simulink model "sim_3_twolink_task_control"  (R2021a)
settings: Solver=VariableStepAuto  StartTime=0.0  StopTime=10.0  RelTol=1e-3
values from neighbouring files (symbols this model uses):
  b1 = 0.01    [sim_params.m]    (also in sim_params_force.m)
  b2 = 0.01    [sim_params.m]    (also in sim_params_force.m)
  D = [zeros(n); eye(n)]    [control_comparison_script.m]    (also in gen_twolink_ss.m = reshape([0.0,0.0,0.0,0.0,0.0,0.0,0.0,0.0],[4,2]))
  g = 9.80665    [sim_params.m]    (also in sim_params_force.m)
  Klqr = lqr(A,B,Q,R)    [control_comparison_script.m]
  Kpp = place(A,B,p)    [control_comparison_script.m]
  L1x = 0.3    [sim_params.m]    (also in sim_params_force.m)
  L1y = 0.050    (= 0.05)    [sim_params.m]    (also in sim_params_force.m)
  L1z = 0.05    [sim_params.m]    (also in sim_params_force.m)
  L2x = 0.15    [sim_params.m]    (also in sim_params_force.m = 0.3)
  L2y = 0.05    [sim_params.m]    (also in sim_params_force.m)
  L2z = 0.05    [sim_params.m]    (also in sim_params_force.m)
  m1 = m1*1.25    [control_comparison_script.m]    (also in sim_params.m = 2.775; sim_params_force.m = 2.775)
  m2 = m2*1.25    [control_comparison_script.m]    (also in sim_params.m = 1.3875; sim_params_force.m = 2.775)
  max_joint_torque1 = 20    [sim_params.m]    (also in sim_params_force.m)
  max_joint_torque2 = 10    [sim_params.m]    (also in sim_params_force.m = 20)
  theta1_0 = 0    [sim_params.m]    (also in sim_params_force.m = 1.57079632679)
  theta1_dot_0 = 0    [sim_params.m]    (also in sim_params_force.m)
  theta2_0 = 0    [sim_params.m]    (also in sim_params_force.m = -1.57079632679)
  theta2_dot_0 = 0    [sim_params.m]    (also in sim_params_force.m)
undefined symbols (not defined in the file or in its folder): Kslide, lambda, Levenberg, Marquardt, phi, sigbuilder_block, X, Y, Z
libraries: sm_lib x11, nesl_utility x10, simulink x8, pid_lib x6, robotmaniplib x3, robotcorelib x1
(part 2 of 2)

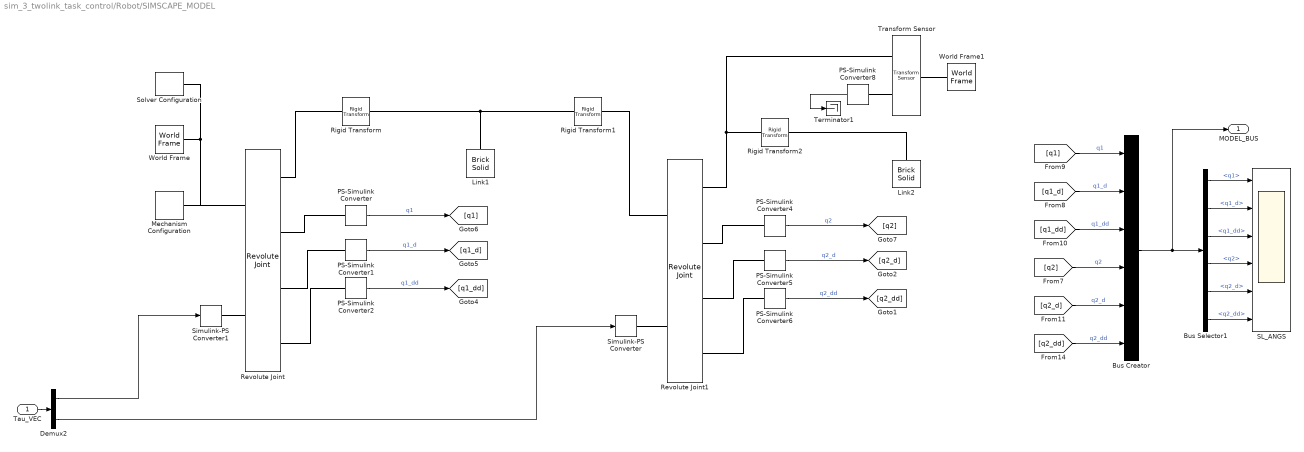
== system sim_3_twolink_task_control/Robot/SIMSCAPE_MODEL ==
  Tau_VEC : Inport
  Bus Creator : BusCreator  Inputs=6
  Bus Selector1 : BusSelector  OutputSignals=q1,q1_d,q1_dd,q2,q2_d,q2_dd
  Demux2 : Demux  Outputs=2
  Link1 : sm_lib/Body Elements/Brick Solid  GraphicAmbientColor=[0.15 0.15 0.15 1.0]  BasedOnType=Density  BrickDimensions=[L1x L1y L1z]  BrickDimensionUnits=m  CenterOfMass=[0 0 0]  CenterOfMassUnits=m  GraphicDiffuseColor=[0.8 0.8 1.0]  Density=density  DensityUnits=kg/m^3  DoExposeReferenceFrame=on  GraphicEmissiveColor=[0.0 0.0 0.0 1.0]  ExportEntireGeometry=off  SerializedFrames=<Frames/>  MarkerShape=Sphere  MarkerSize=10  GraphicType=FromGeometry  InertiaType=CalculateFromGeometry  Mass=1  MassUnits=kg  MomentsOfInertia=[1 1 1]  MomentsOfInertiaUnits=kg*m^2  GraphicOpacity=1.0  ProductsOfInertia=[0 0 0]  ProductsOfInertiaUnits=kg*m^2  GraphicShininess=75  GraphicSpecularColor=[0.5 0.5 0.5 1.0]  GraphicVisPropType=SimpleVisualProperties
  Link2 : sm_lib/Body Elements/Brick Solid  GraphicAmbientColor=[0.15 0.15 0.15 1.0]  BasedOnType=Density  BrickDimensions=[L2x L2y L2z]  BrickDimensionUnits=m  CenterOfMass=[0 0 0]  CenterOfMassUnits=m  GraphicDiffuseColor=[1.0 0.6 1.0]  Density=density  DensityUnits=kg/m^3  DoExposeReferenceFrame=on  GraphicEmissiveColor=[0.0 0.0 0.0 1.0]  ExportEntireGeometry=off  SerializedFrames=<Frames/>  MarkerShape=Sphere  MarkerSize=10  GraphicType=FromGeometry  InertiaType=CalculateFromGeometry  Mass=1  MassUnits=kg  MomentsOfInertia=[1 1 1]  MomentsOfInertiaUnits=kg*m^2  GraphicOpacity=1.0  ProductsOfInertia=[0 0 0]  ProductsOfInertiaUnits=kg*m^2  GraphicShininess=75  GraphicSpecularColor=[0.5 0.5 0.5 1.0]  GraphicVisPropType=SimpleVisualProperties
  Mechanism Configuration : sm_lib/Utilities/Mechanism Configuration  UniformGravity=Constant  GravityVector=[0 -g 0 ]  GravityVectorUnits=m/s^2  GravityUnits=m/s^2  LinearizationDelta=1e-4  JointModeTransitionNonlinearIterations=2
  PS-Simulink Converter : nesl_utility/PS-Simulink Converter  PhysicalDomain=network_engine_domain  SubClassName=ps_output  LeftPortType=input  RightPortType=output  PseudoPeriodic=off  Frequencies=[]  Unit=rad  AffineConversion=off
      settings: SourceProductBaseCode=PW,SS
  PS-Simulink Converter1 : nesl_utility/PS-Simulink Converter  PhysicalDomain=network_engine_domain  SubClassName=ps_output  LeftPortType=input  RightPortType=output  PseudoPeriodic=off  Frequencies=[]  Unit=rad/s  AffineConversion=off
      settings: SourceProductBaseCode=PW,SS
  PS-Simulink Converter2 : nesl_utility/PS-Simulink Converter  PhysicalDomain=network_engine_domain  SubClassName=ps_output  LeftPortType=input  RightPortType=output  PseudoPeriodic=off  Frequencies=[]  Unit=rad/s^2  AffineConversion=off
      settings: SourceProductBaseCode=PW,SS
  PS-Simulink Converter4 : nesl_utility/PS-Simulink Converter  PhysicalDomain=network_engine_domain  SubClassName=ps_output  LeftPortType=input  RightPortType=output  PseudoPeriodic=off  Frequencies=[]  Unit=rad  AffineConversion=off
      settings: SourceProductBaseCode=PW,SS
  PS-Simulink Converter5 : nesl_utility/PS-Simulink Converter  PhysicalDomain=network_engine_domain  SubClassName=ps_output  LeftPortType=input  RightPortType=output  PseudoPeriodic=off  Frequencies=[]  Unit=rad/s  AffineConversion=off
      settings: SourceProductBaseCode=PW,SS
  PS-Simulink Converter6 : nesl_utility/PS-Simulink Converter  PhysicalDomain=network_engine_domain  SubClassName=ps_output  LeftPortType=input  RightPortType=output  PseudoPeriodic=off  Frequencies=[]  Unit=rad/s^2  AffineConversion=off
      settings: SourceProductBaseCode=PW,SS
  PS-Simulink Converter8 : nesl_utility/PS-Simulink Converter  PhysicalDomain=network_engine_domain  SubClassName=ps_output  LeftPortType=input  RightPortType=output  PseudoPeriodic=off  Frequencies=[]  Unit=1  AffineConversion=off
      settings: SourceProductBaseCode=PW,SS
  Revolute Joint : sm_lib/Joints/Revolute Joint  JointMode=Normal  SenseConstraintForce=off  SenseConstraintForceX=off  SenseConstraintForceY=off  SenseConstraintForceZ=off  SenseConstraintTorque=off  SenseConstraintTorqueX=off  SenseConstraintTorqueY=off  SenseConstraintTorqueZ=off  SenseTotalForce=off  SenseTotalForceX=off  SenseTotalForceY=off  SenseTotalForceZ=off  SenseTotalTorque=off  SenseTotalTorqueX=off  SenseTotalTorqueY=off  SenseTotalTorqueZ=off  CompositeWrenchDir=BaseOnFollower  CompositeWrenchFrame=BaseFrame  EquilibriumPosition=0  EquilibriumPositionUnits=deg  SpringStiffness=0  SpringStiffnessUnits=N*m/deg  DampingCoefficient=b1  DampingCoefficientUnits=N*m/(rad/s)  TorqueActuationMode=InputTorque  MotionActuationMode=ComputedMotion  SensePosition=on  SenseVelocity=on  SenseAcceleration=on  SenseTorqueForce=off  SenseLowerLimitTorqueForce=off  SenseUpperLimitTorqueForce=off  LowerLimitSpecify=off  LowerLimitBound=-90  LowerLimitBoundUnits=deg  LowerLimitStiffness=1e4  LowerLimitStiffnessUnits=N*m/deg  LowerLimitDamping=10  LowerLimitDampingUnits=N*m/(deg/s)  LowerLimitTransitionRegionWidth=0.1  LowerLimitTransitionRegionWidthUnits=deg  UpperLimitSpecify=off  UpperLimitBound=90  UpperLimitBoundUnits=deg  UpperLimitStiffness=1e4  UpperLimitStiffnessUnits=N*m/deg  UpperLimitDamping=10  UpperLimitDampingUnits=N*m/(deg/s)  UpperLimitTransitionRegionWidth=0.1  UpperLimitTransitionRegionWidthUnits=deg  PositionTargetSpecify=on  PositionTargetPriority=Low  PositionTargetValue=theta1_0  PositionTargetValueUnits=rad  VelocityTargetSpecify=on  VelocityTargetPriority=High  VelocityTargetValue=theta1_dot_0  VelocityTargetValueUnits=rad/s
      settings: AttributesFormatString=|
      | %<DampingCoefficient>
      | %<PositionTargetValue>
      | %<VelocityTargetValue>
  Revolute Joint1 : sm_lib/Joints/Revolute Joint  JointMode=Normal  SenseConstraintForce=off  SenseConstraintForceX=off  SenseConstraintForceY=off  SenseConstraintForceZ=off  SenseConstraintTorque=off  SenseConstraintTorqueX=off  SenseConstraintTorqueY=off  SenseConstraintTorqueZ=off  SenseTotalForce=off  SenseTotalForceX=off  SenseTotalForceY=off  SenseTotalForceZ=off  SenseTotalTorque=off  SenseTotalTorqueX=off  SenseTotalTorqueY=off  SenseTotalTorqueZ=off  CompositeWrenchDir=BaseOnFollower  CompositeWrenchFrame=FollowerFrame  EquilibriumPosition=0  EquilibriumPositionUnits=deg  SpringStiffness=0  SpringStiffnessUnits=N*m/deg  DampingCoefficient=b2  DampingCoefficientUnits=N*m/(rad/s)  TorqueActuationMode=InputTorque  MotionActuationMode=ComputedMotion  SensePosition=on  SenseVelocity=on  SenseAcceleration=on  SenseTorqueForce=off  SenseLowerLimitTorqueForce=off  SenseUpperLimitTorqueForce=off  LowerLimitSpecify=off  LowerLimitBound=-90  LowerLimitBoundUnits=deg  LowerLimitStiffness=1e4  LowerLimitStiffnessUnits=N*m/deg  LowerLimitDamping=10  LowerLimitDampingUnits=N*m/(deg/s)  LowerLimitTransitionRegionWidth=0.1  LowerLimitTransitionRegionWidthUnits=deg  UpperLimitSpecify=off  UpperLimitBound=90  UpperLimitBoundUnits=deg  UpperLimitStiffness=1e4  UpperLimitStiffnessUnits=N*m/deg  UpperLimitDamping=10  UpperLimitDampingUnits=N*m/(deg/s)  UpperLimitTransitionRegionWidth=0.1  UpperLimitTransitionRegionWidthUnits=deg  PositionTargetSpecify=on  PositionTargetPriority=Low  PositionTargetValue=theta2_0  PositionTargetValueUnits=rad  VelocityTargetSpecify=on  VelocityTargetPriority=High  VelocityTargetValue=theta2_dot_0  VelocityTargetValueUnits=rad/s
      settings: AttributesFormatString=|
      | %<DampingCoefficient>
      | %<PositionTargetValue>
      | %<VelocityTargetValue>
  Rigid Transform : sm_lib/Frames and Transforms/Rigid Transform  TranslationMethod=StandardAxis  TranslationStandardOffset=L1x/2  TranslationLengthUnit=m  TranslationStandardAxis=+X  TranslationCartesianOffset=[0 0 0]  TranslationROffset=0  TranslationROffsetUnits=m  TranslationZOffset=0  TranslationZOffsetUnits=m  TranslationThetaOffset=0  TranslationThetaOffsetUnits=deg  RotationMethod=None  RotationAngleUnits=deg  RotationStandardAxis=+Z  RotationAngle=0.0  RotationArbitraryAxis=[0 0 1]  FollAlignAxisA=+X  BaseAlignAxisA=+Y  FollAlignAxisB=+Y  BaseAlignAxisB=+Z  RotationSequenceAxes=FollowerAxes  RotationSequence=XYX  RotationSequenceAngles=[0 0 0]  RotationSequenceAnglesUnits=deg  RotationMatrix=[1 0 0; 0 1 0; 0 0 1]
  Rigid Transform1 : sm_lib/Frames and Transforms/Rigid Transform  TranslationMethod=StandardAxis  TranslationStandardOffset=L1x/2  TranslationLengthUnit=m  TranslationStandardAxis=+X  TranslationCartesianOffset=[0 0 0]  TranslationROffset=0  TranslationROffsetUnits=m  TranslationZOffset=0  TranslationZOffsetUnits=m  TranslationThetaOffset=0  TranslationThetaOffsetUnits=deg  RotationMethod=None  RotationAngleUnits=deg  RotationStandardAxis=+Z  RotationAngle=0.0  RotationArbitraryAxis=[0 0 1]  FollAlignAxisA=+X  BaseAlignAxisA=+Y  FollAlignAxisB=+Y  BaseAlignAxisB=+Z  RotationSequenceAxes=FollowerAxes  RotationSequence=XYX  RotationSequenceAngles=[0 0 0]  RotationSequenceAnglesUnits=deg  RotationMatrix=[1 0 0; 0 1 0; 0 0 1]
  Rigid Transform2 : sm_lib/Frames and Transforms/Rigid Transform  TranslationMethod=StandardAxis  TranslationStandardOffset=L2x/2  TranslationLengthUnit=m  TranslationStandardAxis=+X  TranslationCartesianOffset=[0 0 0]  TranslationROffset=0  TranslationROffsetUnits=m  TranslationZOffset=0  TranslationZOffsetUnits=m  TranslationThetaOffset=0  TranslationThetaOffsetUnits=deg  RotationMethod=None  RotationAngleUnits=deg  RotationStandardAxis=+Z  RotationAngle=0.0  RotationArbitraryAxis=[0 0 1]  FollAlignAxisA=+X  BaseAlignAxisA=+Y  FollAlignAxisB=+Y  BaseAlignAxisB=+Z  RotationSequenceAxes=FollowerAxes  RotationSequence=XYX  RotationSequenceAngles=[0 0 0]  RotationSequenceAnglesUnits=deg  RotationMatrix=[1 0 0; 0 1 0; 0 0 1]
  SL_ANGS : Scope  NumInputPorts=6
  Simulink-PS Converter : nesl_utility/Simulink-PS Converter  PhysicalDomain=network_engine_domain  SubClassName=ps_input  LeftPortType=input  RightPortType=output  PseudoPeriodic=off  Frequencies=[]  NoiseDistribution=none  NoiseParameters=[]  Unit=N*m  AffineConversion=off  FilteringAndDerivatives=zero  SimscapeFilterOrder=1  InputFilterTimeConstant=0.001  UdotUserProvided=1
      settings: SourceProductBaseCode=PW,SS
  Simulink-PS Converter1 : nesl_utility/Simulink-PS Converter  PhysicalDomain=network_engine_domain  SubClassName=ps_input  LeftPortType=input  RightPortType=output  PseudoPeriodic=off  Frequencies=[]  NoiseDistribution=none  NoiseParameters=[]  Unit=N*m  AffineConversion=off  FilteringAndDerivatives=zero  SimscapeFilterOrder=1  InputFilterTimeConstant=0.001  UdotUserProvided=1
      settings: SourceProductBaseCode=PW,SS
  Solver Configuration : nesl_utility/Solver Configuration  PhysicalDomain=network_engine_domain  SubClassName=solver  LeftPortType=input  RightPortType=generic  Tones=[]  Harmonics=[]  SimulateNoise=off  Profile=off  UseLocalSampling=off  EnableSwitchedLinearOptims=on  FrequencyDomain=off  UseCCode=off  RelTol=0.001  AbsTol=1e-06  MinStep=1e-09  ToWorkspace=off  RevertToSquareIcSolve=off  NumHomotopyIterations=100  PhasorMode=off  PhasorModeNumHarmonics=1  DoDC=off  ResidualTolerance=1e-09  UseLocalSolver=off  LocalSolverChoice=NE_TRAPEZOIDAL_ADVANCER  LocalSolverSampleTime=0.01  DoFixedCost=off  MaxNonlinIter=3  MaxModeIter=2  ComputeImpulses=off  ImpulseIterations=2  LinearAlgebra=Sparse  EquationFormulation=NE_TIME_EF  DelaysMemoryBudget=1024  AutomaticFiltering=off  FilteringTimeConstant=0.001  PartitionStorageMethod=AS_NEEDED  PartitionMemoryBudget=1024  PartitionMethod=FAST
      settings: SourceProductBaseCode=PW,SS
  Terminator1 : Terminator
  Transform Sensor : sm_lib/Frames and Transforms/Transform Sensor  MeasurementFrame=World  SenseAngle=off  SenseAxis=off  SenseAngle1=off  SenseAngle2=off  SenseAngle3=off  SenseQ=off  SenseR=on  SenseOmegaX=off  SenseOmegaY=off  SenseOmegaZ=off  SenseOmega1=off  SenseOmega2=off  SenseOmega3=off  SenseQDot=off  SenseRDot=off  SenseAlphaX=off  SenseAlphaY=off  SenseAlphaZ=off  SenseAlpha1=off  SenseAlpha2=off  SenseAlpha3=off  SenseQDDot=off  SenseRDDot=off  SenseX=off  SenseY=off  SenseZ=off  SenseRad=off  SenseAzim=off  SenseDist=off  SenseInc=off  SenseXDot=off  SenseYDot=off  SenseZDot=off  SenseRadDot=off  SenseAzimDot=off  SenseDistDot=off  SenseIncDot=off  SenseXDDot=off  SenseYDDot=off  SenseZDDot=off  SenseRadDDot=off  SenseAzimDDot=off  SenseDistDDot=off  SenseIncDDot=off
  World Frame : sm_lib/Frames and Transforms/World Frame
  World Frame1 : sm_lib/Frames and Transforms/World Frame
  MODEL_BUS : Outport
  wires:
  PS-Simulink Converter/1 -> [q1]  "q1"
  PS-Simulink Converter2/1 -> [q1_dd]  "q1_dd"
  PS-Simulink Converter1/1 -> [q1_d]  "q1_d"
  Bus Creator/1 -> Bus Selector1/1, MODEL_BUS/1
  PS-Simulink Converter4/1 -> [q2]  "q2"
  PS-Simulink Converter6/1 -> [q2_dd]  "q2_dd"
  PS-Simulink Converter5/1 -> [q2_d]  "q2_d"
  Tau_VEC/1 -> Demux2/1
  Demux2/1 -> Simulink-PS Converter1/1
  Demux2/2 -> Simulink-PS Converter/1
  Bus Selector1/2 -> SL_ANGS/2  "<q1_d>"
  Bus Selector1/5 -> SL_ANGS/5  "<q2_d>"
  Bus Selector1/6 -> SL_ANGS/6  "<q2_dd>"
  Bus Selector1/1 -> SL_ANGS/1  "<q1>"
  Bus Selector1/3 -> SL_ANGS/3  "<q1_dd>"
  [q1_dd] -> Bus Creator/3  "q1_dd"
  [q1] -> Bus Creator/1  "q1"
  [q2] -> Bus Creator/4  "q2"
  [q2_d] -> Bus Creator/5  "q2_d"
  [q1_d] -> Bus Creator/2  "q1_d"
  [q2_dd] -> Bus Creator/6  "q2_dd"
  Bus Selector1/4 -> SL_ANGS/4  "<q2>"
  PS-Simulink Converter8/1 -> Terminator1/1
  connections:
  World Frame/RConn1 -- Revolute Joint/LConn1 -- Mechanism Configuration/RConn1 -- Solver Configuration/RConn1
  Rigid Transform1/LConn1 -- Link1/RConn1 -- Rigid Transform/RConn1
  Revolute Joint/RConn3 -- PS-Simulink Converter1/LConn1
  Revolute Joint/RConn4 -- PS-Simulink Converter2/LConn1
  Rigid Transform/LConn1 -- Revolute Joint/RConn1
  PS-Simulink Converter/LConn1 -- Revolute Joint/RConn2
  Revolute Joint1/LConn1 -- Rigid Transform1/RConn1
  Revolute Joint1/RConn3 -- PS-Simulink Converter5/LConn1
  Revolute Joint1/RConn2 -- PS-Simulink Converter4/LConn1
  Revolute Joint1/RConn4 -- PS-Simulink Converter6/LConn1
  Link2/RConn1 -- Rigid Transform2/RConn1
  Rigid Transform2/LConn1 -- Transform Sensor/RConn1 -- Revolute Joint1/RConn1
  World Frame1/RConn1 -- Transform Sensor/LConn1
  PS-Simulink Converter8/LConn1 -- Transform Sensor/RConn2
  Simulink-PS Converter/RConn1 -- Revolute Joint1/LConn2
  Simulink-PS Converter1/RConn1 -- Revolute Joint/LConn2

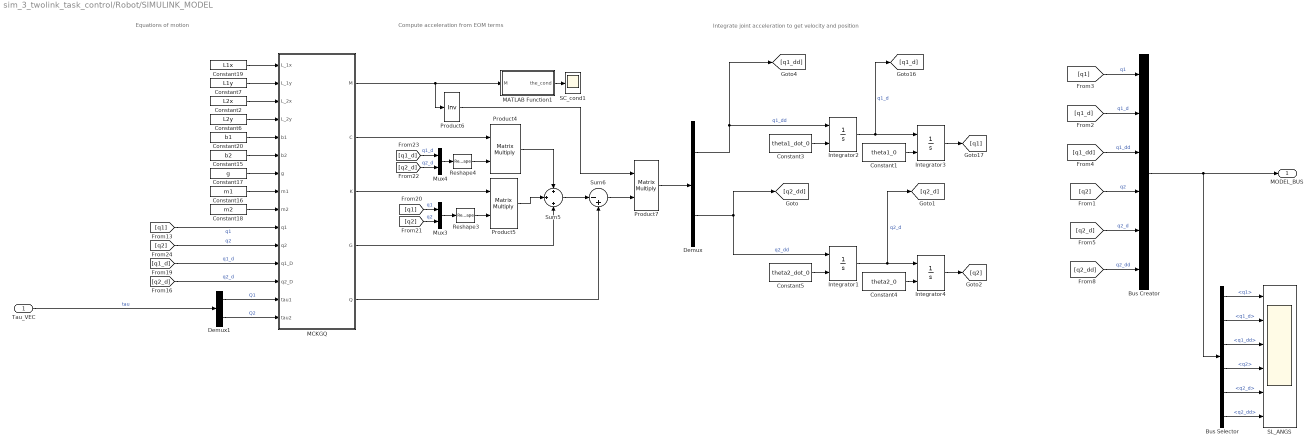
== system sim_3_twolink_task_control/Robot/SIMULINK_MODEL ==
  note: Integrate joint acceleration to get velocity and position
  note: Compute acceleration from EOM terms
  note: Equations of motion
  Tau_VEC : Inport
  Bus Creator : BusCreator  Inputs=6
  Bus Selector : BusSelector  OutputSignals=q1,q1_d,q1_dd,q2,q2_d,q2_dd
  Constant1 : Constant  Value=theta1_0
  Constant15 : Constant  Value=b2
  Constant16 : Constant  Value=m1
  Constant17 : Constant  Value=g
  Constant18 : Constant  Value=m2
  Constant19 : Constant  Value=L1x
  Constant2 : Constant  Value=L2x
  Constant20 : Constant  Value=b1
  Constant3 : Constant  Value=theta1_dot_0
  Constant4 : Constant  Value=theta2_0
  Constant5 : Constant  Value=theta2_dot_0
  Constant6 : Constant  Value=L2y
  Constant7 : Constant  Value=L1y
  Demux : Demux  Outputs=2
  Demux1 : Demux  Outputs=2
  Integrator{1..4} (4 alike) : Integrator  InitialConditionSource=external
  MATLAB Function1 : MATLAB Function  TreatAsAtomicUnit=on
  MCKGQ : MATLAB Function  TreatAsAtomicUnit=on
  Mux3 : Mux  Inputs=2
  Mux4 : Mux  Inputs=2
  Product4 : Product  Multiplication=Matrix(*)
  Product5 : Product  Multiplication=Matrix(*)
  Product6 : Product  Inputs=/  Multiplication=Matrix(*)
  Product7 : Product  Multiplication=Matrix(*)
  Reshape3 : Reshape  OutputDimensionality=Column vector (2-D)
  Reshape4 : Reshape  OutputDimensionality=Column vector (2-D)
  SC_cond1 : Scope
  SL_ANGS : Scope  NumInputPorts=6
  Sum5 : Sum  Inputs=+|+|+
  Sum6 : Sum  Inputs=|-+
  MODEL_BUS : Outport
  wires:
  Bus Creator/1 -> Bus Selector/1, MODEL_BUS/1
  Bus Selector/2 -> SL_ANGS/2  "<q1_d>"
  Bus Selector/3 -> SL_ANGS/3  "<q1_dd>"
  Bus Selector/1 -> SL_ANGS/1  "<q1>"
  Bus Selector/4 -> SL_ANGS/4  "<q2>"
  Bus Selector/6 -> SL_ANGS/6  "<q2_dd>"
  Integrator3/1 -> [q1]
  Integrator2/1 -> [q1_d], Integrator3/1  "q1_d"
  Constant3/1 -> Integrator2/2
  Constant1/1 -> Integrator3/2
  Integrator1/1 -> [q2_d], Integrator4/1  "q2_d"
  Constant4/1 -> Integrator4/2
  Integrator4/1 -> [q2]
  Constant5/1 -> Integrator1/2
  [q1_d] -> Bus Creator/2  "q1_d"
  [q2_d] -> Bus Creator/5  "q2_d"
  [q2] -> Bus Creator/4  "q2"
  [q2_dd] -> Bus Creator/6  "q2_dd"
  [q1] -> Bus Creator/1  "q1"
  [q1_dd] -> Bus Creator/3  "q1_dd"
  Demux/1 -> [q1_dd], Integrator2/1  "q1_dd"
  Demux/2 -> [q2_dd], Integrator1/1  "q2_dd"
  MCKGQ/5(Q) -> Sum6/2
  [q1] -> Mux3/1  "q1"
  Sum6/1 -> Product7/2
  [q2] -> Mux3/2  "q2"
  Sum5/1 -> Sum6/1
  Product4/1 -> Sum5/1
  Constant18/1 -> MCKGQ/9(m2)
  Product5/1 -> Sum5/2
  Demux1/2 -> MCKGQ/15(tau2)  "Q2"
  MCKGQ/3(K) -> Product5/1
  MATLAB Function1/1(the_cond) -> SC_cond1/1
  Product6/1 -> Product7/1
  Constant20/1 -> MCKGQ/5(b1)
  Reshape3/1 -> Product5/2
  [q1] -> MCKGQ/10(q1)  "q1"
  Constant6/1 -> MCKGQ/4(L_2y)
  MCKGQ/4(G) -> Sum5/3
  Constant15/1 -> MCKGQ/6(b2)
  [q1_d] -> MCKGQ/12(q1_D)  "q1_d"
  Constant2/1 -> MCKGQ/3(L_2x)
  Constant19/1 -> MCKGQ/1(L_1x)
  Constant7/1 -> MCKGQ/2(L_1y)
  MCKGQ/2(C) -> Product4/1
  [q1_d] -> Mux4/1  "q1_d"
  Mux3/1 -> Reshape3/1
  Reshape4/1 -> Product4/2
  [q2_d] -> MCKGQ/13(q2_D)  "q2_d"
  [q2_d] -> Mux4/2  "q2_d"
  Demux1/1 -> MCKGQ/14(tau1)  "Q1"
  MCKGQ/1(M) -> MATLAB Function1/1(M), Product6/1
  Mux4/1 -> Reshape4/1
  [q2] -> MCKGQ/11(q2)  "q2"
  Constant17/1 -> MCKGQ/7(g)
  Constant16/1 -> MCKGQ/8(m1)
  Product7/1 -> Demux/1
  Bus Selector/5 -> SL_ANGS/5  "<q2_d>"
  Tau_VEC/1 -> Demux1/1  "tau"

== system sim_3_twolink_task_control/Trajectory/Sinewave command ==
  note: Note: Using derivative blocks without limiters can result in spikes in the signal. Better to manually create the derivative of the signal
  Bus Creator : BusCreator  Inputs=6
  ddx_sin : Sin  Amplitude=-0.45  Frequency=0.25  SampleTime=0  VectorParams1D=off
  ddy_cos : Sin  Amplitude=-0.45  Frequency=0.25  Phase=pi/2  SampleTime=0  VectorParams1D=off
  dx_cos : Sin  Amplitude=0.45  Frequency=0.25  Phase=pi/2  SampleTime=0  VectorParams1D=off
  dy_sin : Sin  Amplitude=-0.45  Frequency=0.25  SampleTime=0  VectorParams1D=off
  x_sin : Sin  Amplitude=0.45  Frequency=0.25  SampleTime=0  VectorParams1D=off
  y_cos : Sin  Amplitude=0.45  Frequency=0.25  Phase=pi/2  SampleTime=0  VectorParams1D=off
  CMD : Outport
  wires:
  Bus Creator/1 -> CMD/1
  y_cos/1 -> Bus Creator/6  "cmd_y"
  ddy_cos/1 -> Bus Creator/2  "cmd_y_dd"
  ddx_sin/1 -> Bus Creator/1  "cmd_x_dd"
  x_sin/1 -> Bus Creator/5  "cmd_x"
  dx_cos/1 -> Bus Creator/3  "cmd_x_d"
  dy_sin/1 -> Bus Creator/4  "cmd_y_d"

== system sim_3_twolink_task_control/Trajectory/Step command ==
  Bus Creator : BusCreator  Inputs=6
  Constant : Constant  Value=0
  Constant1 : Constant  Value=0
  Discrete Derivative : simulink/Discrete/Discrete Derivative  gainval=1.0  ICPrevScaledInput=0.0  OutMin=[]  OutMax=[]  OutDataType=fixdt(1, 16)  OutScaling=2^-10  DoSatur=off
  Discrete Derivative1 : simulink/Discrete/Discrete Derivative  gainval=1.0  ICPrevScaledInput=0.0  OutMin=[]  OutMax=[]  OutDataType=fixdt(1, 16)  OutScaling=2^-10  DoSatur=off
  Joint commands : Subsystem  Tag=STV Subsys  LoadFcn=sigbuilder_block('load');  StartFcn=sigbuilder_block('start');  StopFcn=sigbuilder_block('stop');  ClipboardFcn=sigbuilder_block('clipboard');  mask(Sigbuilder block){tuvar=[0:10]}
      mask help: Simulink:masks:SigbuilderBlock_MD
      mask init:
      | if ~strcmp(get_param(bdroot(gcbh),'SimulationStatus'),'stopped') tuvar = sigbuilder_block('maskInit'); end
      settings: CopyFcn=sigbuilder_block('copy');  DeleteFcn=sigbuilder_block('delete');  ModelCloseFcn=sigbuilder_block('modelClose');  PreSaveFcn=sigbuilder_block('preSave');  PauseFcn=sigbuilder_block('pause');  ContinueFcn=sigbuilder_block('continue');  NameChangeFcn=sigbuilder_block('namechange');  OpenFcn=sigbuilder_block('open',[4.8 4.8 1142.4 586.8 ]);  CloseFcn=sigbuilder_block('close');
      mask Display: plot(0, 0, 100, 100,[2, 2, 32, 32, 2], [68, 8, 8, 68, 68],[32, 2], [38, 38], [32, 19, 2],[53, 60, 44], [32, 17, 17, 2],[16, 16, 31, 31]);txt = getActiveGroup(gcbh);text(2, 100, txt,'verticalAlignment', 'top');
  Scope : Scope
  CMD : Outport
  wires:
  Bus Creator/1 -> CMD/1
  Discrete Derivative1/1 -> Bus Creator/4  "cmd_y_d"
  Discrete Derivative/1 -> Bus Creator/3, Scope/1  "cmd_x_d"
  Constant/1 -> Bus Creator/1  "cmd_x_dd"
  Constant1/1 -> Bus Creator/2  "cmd_y_dd"
  Joint commands/2(cmd_y) -> Discrete Derivative1/1, Bus Creator/6  "cmd_y"
  Joint commands/1(cmd_x) -> Discrete Derivative/1, Bus Creator/5  "cmd_x"

== system sim_3_twolink_task_control/Trajectory/ramp command ==
  Bus Creator : BusCreator  Inputs=6
  Constant{,1..3} (4 alike) : Constant  Value=0
  Ramp : simulink/Sources/Ramp  slope=0.15/15  start=0  InitialOutput=0.2
  Ramp1 : simulink/Sources/Ramp  slope=0.15/15  start=0  InitialOutput=0.2
  CMD : Outport
  wires:
  Bus Creator/1 -> CMD/1
  Ramp1/1 -> Bus Creator/6  "cmd_y"
  Constant1/1 -> Bus Creator/2  "cmd_y_dd"
  Constant/1 -> Bus Creator/1  "cmd_x_dd"
  Ramp/1 -> Bus Creator/5  "cmd_x"
  Constant2/1 -> Bus Creator/3  "cmd_x_d"
  Constant3/1 -> Bus Creator/4  "cmd_y_d"

== system sim_3_twolink_task_control/Controller/Inverse Dynamics control /FeedForward terms ==
  C : Inport
  K : Inport  Port=2
  G : Inport  Port=3
  q : Inport  Port=4
  q_d : Inport  Port=5
  q_dd : Inport  Port=6
  M : Inport  Port=7
  F : Inport  Port=8
  Product : Product  Multiplication=Matrix(*)
  Product2 : Product  Multiplication=Matrix(*)
  Product3 : Product  Multiplication=Matrix(*)
  Scope : Scope
  Sum : Sum  Inputs=+|+|+|+
  Terminator : Terminator
  Q : Outport
  wires:
  K/1 -> Product/1
  Product/1 -> Sum/3
  Product2/1 -> Sum/1
  Sum/1 -> Q/1
  C/1 -> Product3/1
  Product3/1 -> Sum/2
  M/1 -> Product2/1
  q_dd/1 -> Product2/2
  q/1 -> Product/2
  q_d/1 -> Product3/2
  F/1 -> Terminator/1
  G/1 -> Scope/1, Sum/4

== system sim_3_twolink_task_control/Controller/Inverse Dynamics control /Saturate Inputs ==
  inp : Inport
  Demux : Demux  Outputs=2
  Mux : Mux  Inputs=2
  Saturate Gripper Force : Saturate  UpperLimit=max_joint_torque2  LowerLimit=-max_joint_torque2
  Saturate Joint Torques : Saturate  UpperLimit=max_joint_torque1  LowerLimit=-max_joint_torque1
  sat : Outport  VectorParamsAs1DForOutWhenUnconnected=off
  wires:
  Saturate Joint Torques/1 -> Mux/1
  Demux/1 -> Saturate Joint Torques/1
  Mux/1 -> sat/1
  Saturate Gripper Force/1 -> Mux/2
  inp/1 -> Demux/1
  Demux/2 -> Saturate Gripper Force/1

== system sim_3_twolink_task_control/Controller/PID Control/Saturate Inputs ==
  inp : Inport
  Demux : Demux  Outputs=2
  Mux : Mux  Inputs=2
  Saturate Gripper Force : Saturate  UpperLimit=max_joint_torque2  LowerLimit=-max_joint_torque2
  Saturate Joint Torques : Saturate  UpperLimit=max_joint_torque1  LowerLimit=-max_joint_torque1
  sat : Outport  VectorParamsAs1DForOutWhenUnconnected=off
  wires:
  Saturate Joint Torques/1 -> Mux/1
  Demux/1 -> Saturate Joint Torques/1
  Mux/1 -> sat/1
  Saturate Gripper Force/1 -> Mux/2
  inp/1 -> Demux/1
  Demux/2 -> Saturate Gripper Force/1

== system sim_3_twolink_task_control/Trajectory/Step command/Joint commands ==
  Demux : Demux  Tag=STV Demux  Outputs=2
      settings: DisplayOption=none
  FromWs : FromWorkspace  Tag=STV FromWs  VariableName=tuvar
      SigBuilderData=|
      | common.afterFinalStr = 'Extrapolate'
      | common.sampleTime = 0
      | dataSet(1).timeRange = [0 1000]
      | dataSet(1).name = 'PULSES_SMALL'
      | dataSet(2).timeRange = [0 1000]
      | dataSet(2).name = 'ZERO'
      | dataSet(3).timeRange = [0 1000]
      | dataSet(3).name = 'PULSES_BIG'
      | dataSet(4).timeRange = [0 1000]
      | dataSet(4).name = 'PULSES_SMALL1'
      | sbobj.Groups(1).Name = 'PULSES_SMALL'
      | sbobj.Groups(1).Signals(1).Name = 'cmd_x'
      | sbobj.Groups(1).Signals(1).XData = [0 2.4 2.4 5.05 8.1 8.1 1000]
      | sbobj.Groups(1).Signals(1).YData = [0.2 0.2 0.299 0.299 0.299 0.2 0.2]
      | sbobj.Groups(1).Signals(2).Name = 'cmd_y'
      | sbobj.Groups(1).Signals(2).XData = [0 2.4 2.4 5.05 8.1 8.1 1000]
      | sbobj.Groups(1).Signals(2).YData = [0.2 0.2 0.299 0.299 0.299 0.2 0.2]
      | sbobj.Groups(1).TimeRange = [0 1000]
      | sbobj.Groups(2).Name = 'ZERO'
      | sbobj.Groups(2).Signals(1).Name = 'cmd_x'
      | sbobj.Groups(2).Signals(1).XData = [0 500 500 1000]
      | sbobj.Groups(2).Signals(1).YData = [0 0 1 1]
      | sbobj.Groups(2).Signals(2).Name = 'cmd_y'
      | sbobj.Groups(2).Signals(2).XData = [0 1000]
      | sbobj.Groups(2).Signals(2).YData = [0 0]
      | sbobj.Groups(2).TimeRange = [0 1000]
      | sbobj.Groups(3).Name = 'PULSES_BIG'
      | sbobj.Groups(3).Signals(1).Name = 'cmd_x'
      | sbobj.Groups(3).Signals(1).XData = [0 500 500 1000]
      | sbobj.Groups(3).Signals(1).YData = [0 0 1 1]
      | sbobj.Groups(3).Signals(2).Name = 'cmd_y'
      | sbobj.Groups(3).Signals(2).XData = [0 1000]
      | sbobj.Groups(3).Signals(2).YData = [0 0]
      | sbobj.Groups(3).TimeRange = [0 1000]
      | sbobj.Groups(4).Name = 'PULSES_SMALL1'
      | sbobj.Groups(4).Signals(1).Name = 'cmd_x'
      | sbobj.Groups(4).Signals(1).XData = [0 500 500 1000]
      | sbobj.Groups(4).Signals(1).YData = [0 0 1 1]
      | sbobj.Groups(4).Signals(2).Name = 'cmd_y'
      | sbobj.Groups(4).Signals(2).XData = [0 1000]
      | sbobj.Groups(4).Signals(2).YData = [0 0]
      | sbobj.Groups(4).TimeRange = [0 1000]
  cmd_x : Outport  Tag=STV Outport
  cmd_y : Outport  Tag=STV Outport  Port=2
  wires:
  FromWs/1 -> Demux/1
  Demux/1 -> cmd_x/1
  Demux/2 -> cmd_y/1

== matlab function sim_3_twolink_task_control/Controller/PD-gravity Control /Gravity compensation ==
  data: L_1x input; G output; L_2x input; g input; m1 input; m2 input; q1 input; q2 input
function G = G_compensation(L_1x,L_2x,g,m1,m2,q1,q2)
%#codegen

%    This function was generated by the Symbolic Math Toolbox version 8.7.
%    01-Jun-2022 14:38:05

G = [(g.*(L_2x.*m2.*cos(q1+q2)+L_1x.*m1.*cos(q1)+L_1x.*m2.*cos(q1).*2.0))./2.0;(L_2x.*g.*m2.*cos(q1+q2))./2.0];

== matlab function sim_3_twolink_task_control/Inverse Kinmatics/IK/Inverse Kinematics ==
  data: x input; q1 output; y input; L1 input; L2 input; q2 output
function [q1, q2]= ik_rr(x,y,L1,L2)
%IK_RR 


tmp = (x^2+y^2-L1^2-L2^2)/(2*L1*L2);
if abs(tmp-1)<0.0001
    tmp = 1;
end

if abs(tmp)>1
    q2=0;
else
    q2 = acos(tmp);
    if isnan(q2) || isinf(q2) || ~isreal(q2)
        q2 = 0;
    end
end

q1 = atan2(y,x)-atan2(L2*sin(q2), L1+L2*cos(q2));
if isnan(q1) || isinf(q1) || ~isreal(q1)
    q1 = 0;
end

== matlab function sim_3_twolink_task_control/Forward Kinmatics/Forward Kinematics ==
  data: L_1 input; XE output; L_2 input; theta_1 input; theta_2 input; YE output
function [XE,YE] = FK(L_1,L_2,theta_1,theta_2)

XE = L_2.*cos(theta_1+theta_2)+L_1.*cos(theta_1);
if nargout > 1
    YE = L_2.*sin(theta_1+theta_2)+L_1.*sin(theta_1);
end

== matlab function sim_3_twolink_task_control/Controller/Incremental sliding mode Control/MATLAB Function ==
  data: S input; w output; phi input
function w = sat_sm(S, phi)
    w = sign(S);
    if abs(S(1))<=phi(1)
        w(1) = S(1)/phi(1);
    end
    if abs(S(2))<=phi(2)
        w(2) = S(2)/phi(2);
    end

== matlab function sim_3_twolink_task_control/Controller/Pole Placement+D Control/disturbance_terms ==
  data: L_1x input; d output; L_2x input; g input; m1 input; m2 input; q1 input; q2 input; q1_D input; q2_D input; q1_DD input; q2_DD input
function d = disturbance_terms(L_1x,L_2x,g,m1,m2,q1,q2,q1_D,q2_D,q1_DD,q2_DD)
%#codegen

%    This function was generated by the Symbolic Math Toolbox version 8.7.
%    10-Jun-2022 15:47:18

d = [(g.*(L_2x.*m2.*cos(q1+q2)+L_1x.*m1.*cos(q1)+L_1x.*m2.*cos(q1).*2.0))./2.0+(L_2x.*m2.*q2_DD.*(L_2x+L_1x.*cos(q2).*2.0))./4.0-(L_1x.*L_2x.*m2.*q2_D.^2.*sin(q2))./2.0+L_1x.*L_2x.*m2.*q1_DD.*cos(q2)-L_1x.*L_2x.*m2.*q1_D.*q2_D.*sin(q2);(L_2x.*g.*m2.*cos(q1+q2))./2.0+(L_2x.*m2.*q1_DD.*(L_2x+L_1x.*cos(q2).*2.0))./4.0+(L_1x.*L_2x.*m2.*q1_D.^2.*sin(q2))./2.0];

== matlab function sim_3_twolink_task_control/Inverse Kinmatics/Forward Kinmatics/Forward Kinematics ==
  data: L_1 input; XE output; L_2 input; theta_1 input; theta_2 input; YE output
function [XE,YE] = FK(L_1,L_2,theta_1,theta_2)

XE = L_2.*cos(theta_1+theta_2)+L_1.*cos(theta_1);
if nargout > 1
    YE = L_2.*sin(theta_1+theta_2)+L_1.*sin(theta_1);
end

== matlab function sim_3_twolink_task_control/Robot/SIMULINK_MODEL/MCKGQ ==
  data: L_1x input; M output; L_1y input; L_2x input; L_2y input; b1 input; b2 input; g input; m1 input; m2 input; q1 input; q2 input; q1_D input; q2_D input; tau1 input; tau2 input; C output; K output; G output; Q output
function [M,C,K,G,Q] = MCKGQ(L_1x,L_1y,L_2x,L_2y,b1,b2,g,m1,m2,q1,q2,q1_D,q2_D,tau1,tau2)
%#codegen

%    This function was generated by the Symbolic Math Toolbox version 8.7.
%    30-May-2022 13:59:37

M = reshape([(L_1x.^2.*m1)./3.0+L_1x.^2.*m2+(L_1y.^2.*m1)./1.2e+1+(L_2x.^2.*m2)./4.0+L_1x.*L_2x.*m2.*cos(q2),(L_2x.*m2.*(L_2x+L_1x.*cos(q2).*2.0))./4.0,(L_2x.*m2.*(L_2x+L_1x.*cos(q2).*2.0))./4.0,(m2.*(L_2x.^2.*4.0+L_2y.^2))./1.2e+1],[2,2]);
if nargout > 1
    C = reshape([-L_1x.*L_2x.*m2.*q2_D.*sin(q2),(L_1x.*L_2x.*m2.*q1_D.*sin(q2))./2.0,L_1x.*L_2x.*m2.*q2_D.*sin(q2).*(-1.0./2.0),0.0],[2,2]);
end
if nargout > 2
    K = reshape([0.0,0.0,0.0,0.0],[2,2]);
end
if nargout > 3
    G = [(g.*(L_2x.*m2.*cos(q1+q2)+L_1x.*m1.*cos(q1)+L_1x.*m2.*cos(q1).*2.0))./2.0;(L_2x.*g.*m2.*cos(q1+q2))./2.0];
end
if nargout > 4
    Q = [tau1-b1.*q1_D;tau2-b2.*q2_D];
end

== matlab function sim_3_twolink_task_control/Robot/SIMULINK_MODEL/MATLAB Function1 ==
  data: M input; the_cond output
function the_cond = COND(M)
%#codegen

the_cond = cond(M);

end

== matlab function sim_3_twolink_task_control/Controller/LQR+D Control/disturbance_terms ==
  data: L_1x input; d output; L_2x input; g input; m1 input; m2 input; q1 input; q2 input; q1_D input; q2_D input; q1_DD input; q2_DD input
function d = disturbance_terms(L_1x,L_2x,g,m1,m2,q1,q2,q1_D,q2_D,q1_DD,q2_DD)
%#codegen

%    This function was generated by the Symbolic Math Toolbox version 8.7.
%    10-Jun-2022 15:47:18

d = [(g.*(L_2x.*m2.*cos(q1+q2)+L_1x.*m1.*cos(q1)+L_1x.*m2.*cos(q1).*2.0))./2.0+(L_2x.*m2.*q2_DD.*(L_2x+L_1x.*cos(q2).*2.0))./4.0-(L_1x.*L_2x.*m2.*q2_D.^2.*sin(q2))./2.0+L_1x.*L_2x.*m2.*q1_DD.*cos(q2)-L_1x.*L_2x.*m2.*q1_D.*q2_D.*sin(q2);(L_2x.*g.*m2.*cos(q1+q2))./2.0+(L_2x.*m2.*q1_DD.*(L_2x+L_1x.*cos(q2).*2.0))./4.0+(L_1x.*L_2x.*m2.*q1_D.^2.*sin(q2))./2.0];

== matlab function sim_3_twolink_task_control/Controller/Inverse Dynamics control /MCKGQ ==
  data: L_1x input; M output; L_1y input; L_2x input; L_2y input; b1 input; b2 input; g input; m1 input; m2 input; q1 input; q2 input; q1_D input; q2_D input; tau1 input; tau2 input; C output; K output; G output; Q output
function [M,C,K,G,Q] = MCKGQ(L_1x,L_1y,L_2x,L_2y,b1,b2,g,m1,m2,q1,q2,q1_D,q2_D,tau1,tau2)
%#codegen

%    This function was generated by the Symbolic Math Toolbox version 8.7.
%    30-May-2022 13:59:37

M = reshape([(L_1x.^2.*m1)./3.0+L_1x.^2.*m2+(L_1y.^2.*m1)./1.2e+1+(L_2x.^2.*m2)./4.0+L_1x.*L_2x.*m2.*cos(q2),(L_2x.*m2.*(L_2x+L_1x.*cos(q2).*2.0))./4.0,(L_2x.*m2.*(L_2x+L_1x.*cos(q2).*2.0))./4.0,(m2.*(L_2x.^2.*4.0+L_2y.^2))./1.2e+1],[2,2]);
if nargout > 1
    C = reshape([-L_1x.*L_2x.*m2.*q2_D.*sin(q2),(L_1x.*L_2x.*m2.*q1_D.*sin(q2))./2.0,L_1x.*L_2x.*m2.*q2_D.*sin(q2).*(-1.0./2.0),0.0],[2,2]);
end
if nargout > 2
    K = reshape([0.0,0.0,0.0,0.0],[2,2]);
end
if nargout > 3
    G = [(g.*(L_2x.*m2.*cos(q1+q2)+L_1x.*m1.*cos(q1)+L_1x.*m2.*cos(q1).*2.0))./2.0;(L_2x.*g.*m2.*cos(q1+q2))./2.0];
end
if nargout > 4
    Q = [tau1-b1.*q1_D;tau2-b2.*q2_D];
end
